simulink model "pardoWrite"  (R2024b)
settings: Solver=VariableStepAuto  StartTime=0.0  StopTime=10.0  RelTol=1e-3
settings Model: Creator=ryandavis  LastModifiedBy=ryandavis

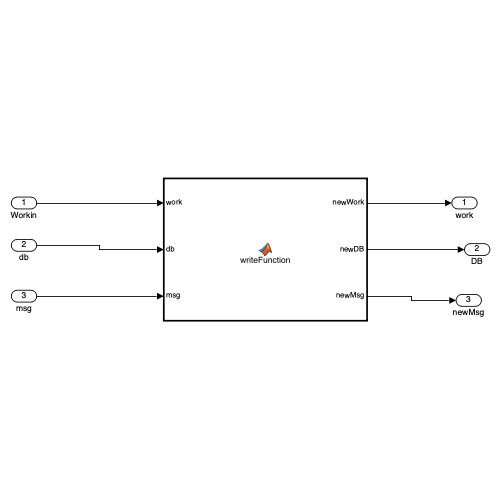
[thumbnail: Simulink's stored preview of the top-level diagram]
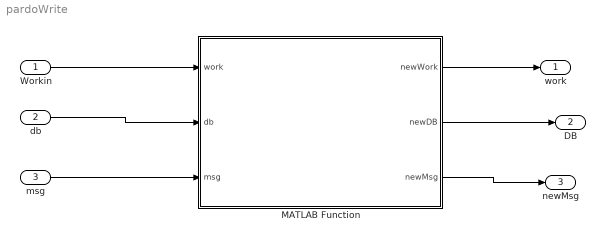
== system pardoWrite ==
  Workin : Inport
  db : Inport  Port=2
  msg : Inport  Port=3
  MATLAB Function : MATLAB Function  TreatAsAtomicUnit=on
  work : Outport
  DB : Outport  Port=2
  newMsg : Outport  Port=3
  wires:
  Workin/1 -> MATLAB Function/1(work)
  MATLAB Function/1(newWork) -> work/1
  MATLAB Function/2(newDB) -> DB/1
  db/1 -> MATLAB Function/2(db)
  msg/1 -> MATLAB Function/3(msg)
  MATLAB Function/3(newMsg) -> newMsg/1

== matlab function pardoWrite/MATLAB Function ==
  data: work input; newWork output; newDB output; db input; msg input; newMsg output
function [newWork, newDB, newMsg] = writeFunction(work, db, msg)
    workNY = 3;
    dbNY = 1;
    msgNY = 2;
    
    workLA = 4;
    dbLA = 1;
    msgLA = 2;

    newWork = work + workNY + workLA;
    newDB = db + dbNY + dbLA;
    newMsg = msg + msgNY + msgLA;
end
